simulink model "Lab8"  (R2015a)
settings: Solver=ode45  StartTime=0.0  StopTime=40  RelTol=1e-3
undefined symbols (not defined in the file or in its folder): currentCFG_Lab8_UB, fdesignblkfcn, gcbh, UB
libraries: dspstat3 x2, gtecHighspeedLib x1, gUSBamplib x1
settings Model: Creator=circuit  LastModifiedBy=circuit

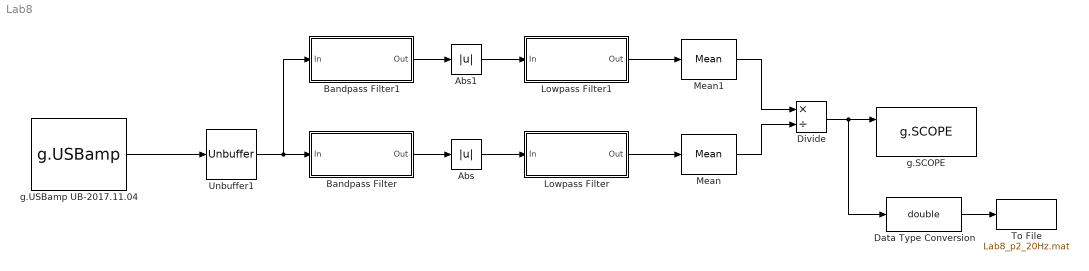
== system Lab8 ==
  Abs : Abs
  Abs1 : Abs
  Bandpass Filter : Subsystem  DialogController=fdesignblkfcn  InitFcn=fdesignblkfcn(gcbh, {'InitFcn'});  mask(Bandpass Filter){}
      mask help: Design a bandpass filter
      settings: CopyFcn=fdesignblkfcn(gcbh, {'CopyFcn'});
      mask Help: helpview(mapfilelocation('dsp'), 'dspbandpassfilter');
      mask Display: disp('Bandpass');
  Bandpass Filter1 : Subsystem  DialogController=fdesignblkfcn  InitFcn=fdesignblkfcn(gcbh, {'InitFcn'});  mask(Bandpass Filter){}
      mask help: Design a bandpass filter
      settings: CopyFcn=fdesignblkfcn(gcbh, {'CopyFcn'});
      mask Help: helpview(mapfilelocation('dsp'), 'dspbandpassfilter');
      mask Display: disp('Bandpass');
  Data Type Conversion : DataTypeConversion  OutDataTypeStr=double
  Divide : Product  Inputs=*/
  Lowpass Filter : Subsystem  DialogController=fdesignblkfcn  InitFcn=fdesignblkfcn(gcbh, {'InitFcn'});  mask(Lowpass Filter){}
      mask help: Design a lowpass filter
      settings: CopyFcn=fdesignblkfcn(gcbh, {'CopyFcn'});
      mask Help: helpview(mapfilelocation('dsp'), 'dsplowpassfilter');
      mask Display: disp('Lowpass')
  Lowpass Filter1 : Subsystem  DialogController=fdesignblkfcn  InitFcn=fdesignblkfcn(gcbh, {'InitFcn'});  mask(Lowpass Filter){}
      mask help: Design a lowpass filter
      settings: CopyFcn=fdesignblkfcn(gcbh, {'CopyFcn'});
      mask Help: helpview(mapfilelocation('dsp'), 'dsplowpassfilter');
      mask Display: disp('Lowpass')
  Mean : dspstat3/Mean  run=off  reset_popup=None  InputProcessing=Columns as channels (frame based)  directionMode=Each row  dimension=1  treatSBRowAsCol=off  roiEnable=off  roiType=Rectangles  roiPortion=Entire ROI  roiOutput=Individual statistics for each ROI  roiFlag=off  outputDataTypeStr=Inherit: Same as accumulator  outputLastDataTypeStr=Inherit: Same as accumulator  outputMin=[]  outputMax=[]  roundingMode=Floor  overflowMode=off
  Mean1 : dspstat3/Mean  run=off  reset_popup=None  InputProcessing=Columns as channels (frame based)  directionMode=Each row  dimension=1  treatSBRowAsCol=off  roiEnable=off  roiType=Rectangles  roiPortion=Entire ROI  roiOutput=Individual statistics for each ROI  roiFlag=off  outputDataTypeStr=Inherit: Same as accumulator  outputLastDataTypeStr=Inherit: Same as accumulator  outputMin=[]  outputMax=[]  roundingMode=Floor  overflowMode=off
  To File : ToFile  Filename=Lab8_p2_20Hz.mat
  Unbuffer1 : Unbuffer  SampleBasedProcessing=Same as frame based
  g.SCOPE : gtecHighspeedLib/g.SCOPE
  g.USBamp UB-2017.11.04 : gUSBamplib/g.USBamp  cfg=currentCFG_Lab8_UB-2017.11.04.cfg  snr=UB-2017.11.04
  wires:
  g.USBamp UB-2017.11.04/1 -> Unbuffer1/1
  Data Type Conversion/1 -> To File/1
  Bandpass Filter/1(Out) -> Abs/1
  Abs/1 -> Lowpass Filter/1(In)
  Lowpass Filter/1(Out) -> Mean/1
  Bandpass Filter1/1(Out) -> Abs1/1
  Abs1/1 -> Lowpass Filter1/1(In)
  Lowpass Filter1/1(Out) -> Mean1/1
  Unbuffer1/1 -> Bandpass Filter1/1(In), Bandpass Filter/1(In)
  Mean1/1 -> Divide/1
  Mean/1 -> Divide/2
  Divide/1 -> Data Type Conversion/1, g.SCOPE/1

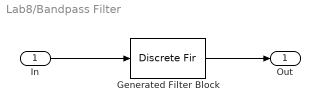
== system Lab8/Bandpass Filter ==
  In : Inport
  Generated Filter Block : DiscreteFir  Tag=BlockMethodSubSystem  Coefficients=[-9.707325903234668e-20 -1.4547940133680366e-05 -3.8949317559313134e-06 3.6026346384903206e-05 8.0448494737471273e-05 8.967465436443488e-05 3.7220119308981178e-05 -6.5501979123452491e-05 -0.00016597972781469807 -0.00019559147132576537 -0.00011199693878070027 6.5444622755014026e-05 0.00025203975411325575 0.00033537692656571258 0.00023929136553389044 -2.0493259905462968e-05 -0.00032560178590533242 -0.00050507650455621823 -0.0004277162252905762 -8.8528512668217872e-05 0.0003643080739927531 0.00068914948173672778 0.0006767539903635159 0.00027840235241952403 -0.00033958389430201825 -0.00085892159233023652 -0.00097081207789280141 -0.00055532890114523049 0.00022376136587924606 0.00097550797468224401 0.0012763435998424657 0.00090701727469001019 -1.3887637912025664e-18 -0.00099759244566786465 -0.0015439245373024095 -0.0012977059666992453 -0.00032731489556745731 0.00089308971486456654 0.0017161379540980648 0.0016685062324890048 0.00072466657028648004 -0.00065239693882807395 -0.001740671604790883 -0.0019445085536974286 -0.0011269354766907974 0.00030000334130668839 0.0015865019927581324 0.0020486066922622411 0.0014425109771110652 9.9042847240027109e-05 -0.0012597855387530821 -0.001920268606546659 -0.0015666716493755515 -0.00044075704605277499 0.00081544817158235193 0.0015359045645405192 0.0014020487983387941 0.0005935236471211751 -0.00036069024969694979 -0.00092644253770405118 -0.00088309532029252587 -0.00041873516814926295 4.776277178711424e-05 0.00018752915637505508 -6.5524449846833991e-19 -0.00020174488467054801 -5.5280066024992317e-05 0.00052141907608394336 0.0011832002845955873 0.0013357303032482299 0.00055968338192752905 -0.00099134229557729038 -0.0025212044943446008 -0.0029741453706790088 -0.0017007993626627198 0.0009904502538131809 0.003794183319845532 0.0050136260215938302 0.0035472478609025683 -0.00030087848750407051 -0.0047297848643821708 -0.0072531961505064354 -0.0060683103227048207 -0.0012403120709677583 0.0050386817714201193 0.0094078452364920653 0.0091185003577514967 0.0037027406841594478 -0.0044591076744620213 -0.0111389632161377 -0.0124394403636592 -0.0070342200886887255 0.0028035980128727342 0.012098431295184965 0.015680955581780381 0.011048464396676115 -1.5748967504052466e-17 -0.0119803203801235 -0.018439990783413261 -0.015432981404860749 -0.0038809415095607193 0.010572188456240368 0.02031262760549268 0.019777907844435092 0.008617426673178389 -0.0077973328141100204 -0.020951765911774806 -0.023622932270838583 -0.013850965299664677 0.0037402480337457382 0.020121480748256981 0.026516109949488494 0.019122696977364507 0.0013501128300229541 -0.017739032099786174 -0.028075943326947808 -0.023927330542281085 -0.0070812382767018274 0.013897069150475779 0.028047071501226335 0.027777174728241 0.012960135759938648 -0.0088615165124812691 -0.026340528101279799 -0.030266721377044666 -0.01845284220300266 0.0030444728151259146 0.023051734501646579 0.031127815551427521 0.023051734501646579 0.0030444728151259146 -0.01845284220300266 -0.030266721377044666 -0.026340528101279799 -0.0088615165124812691 0.012960135759938648 0.027777174728241 0.028047071501226335 0.013897069150475779 -0.0070812382767018274 -0.023927330542281085 -0.028075943326947808 -0.017739032099786174 0.0013501128300229541 0.019122696977364507 0.026516109949488494 0.020121480748256981 0.0037402480337457382 -0.013850965299664677 -0.023622932270838583 -0.020951765911774806 -0.0077973328141100204 0.008617426673178389 0.019777907844435092 0.02031262760549268 0.010572188456240368 -0.0038809415095607193 -0.015432981404860749 -0.018439990783413261 -0.0119803203801235 -1.5748967504052466e-17 0.011048464396676115 0.015680955581780381 0.012098431295184965 0.0028035980128727342 -0.0070342200886887255 -0.0124394403636592 -0.0111389632161377 -0.0044591076744620213 0.0037027406841594478 0.0091185003577514967 0.0094078452364920653 0.0050386817714201193 -0.0012403120709677583 -0.0060683103227048207 -0.0072531961505064354 -0.0047297848643821708 -0.00030087848750407051 0.0035472478609025683 ...(+1800 chars)]  InputProcessing=Columns as channels (frame based)
  Out : Outport
  wires:
  In/1 -> Generated Filter Block/1
  Generated Filter Block/1 -> Out/1

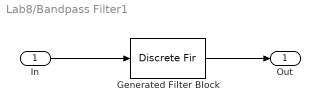
== system Lab8/Bandpass Filter1 ==
  In : Inport
  Generated Filter Block : DiscreteFir  Tag=BlockMethodSubSystem  Coefficients=[-1.5051096604374551e-18 -1.7315578160519554e-05 -2.2076592085780425e-05 -5.9277570357802236e-06 3.1389101425903213e-05 8.0816571350543964e-05 0.00012575429528274929 0.00014660285843847034 0.00012703399144143099 6.0301569398176467e-05 -4.6350086138402551e-05 -0.00017086650482735775 -0.0002800485001784454 -0.00033741029355496003 -0.00031362456545468598 -0.00019687808908326084 1.4905324401675337e-19 0.00023837594061658335 0.00046005735672647371 0.00060042917678830088 0.00060581554561807362 0.00045069373740795371 0.00014970350763937406 -0.00023988567888102094 -0.00062746234129258172 -0.00090922283468534656 -0.00099499177096056251 -0.00083498939690683494 -0.00043891889687715094 0.00011904202866567846 0.00071252172555333847 0.0011911226079923925 0.0014183952150465735 0.001310068670967178 0.00086189939415892843 0.0001583601107287249 -0.00064204422568400602 -0.0013428446473082586 -0.0017588812305126885 -0.0017662193847963654 -0.0013389945473798743 -0.00056213850641189137 0.00038505076969768689 0.0012716803113296596 0.0018740046664499222 0.0020347202706273528 0.0017064630006349019 0.00096686055046356085 4.7167813563242699e-19 -0.00095150144935152734 -0.0016511238977470455 -0.001931911061604685 -0.0017407731856561217 -0.0011507533051109246 -0.00033747433997506014 0.00047352502161691326 0.0010730699308501433 0.0013283913613479736 0.0012186513371829463 0.00083492833043168199 0.00034456292399080029 -6.8898475371502717e-05 -0.00027072084845249062 -0.00022320519157696217 1.0159490207952821e-17 0.0002401253570538214 0.00031332910165891191 8.5794034283249131e-05 -0.00046165678875068381 -0.0012037865562195325 -0.0018909823660554306 -0.0022187667634999313 -0.0019296252281738834 -0.00091693994760927281 0.00070387814007949164 0.0025859232729928535 0.0042158244117606637 0.005044023287598759 0.004649160935888701 0.0028905299566458318 -6.1862575527630841e-18 -0.0034232189366494221 -0.0065271566561753121 -0.0084122000165389298 -0.0083789297148803999 -0.0061525939479847936 -0.0020170867219165564 0.0031904703930140648 0.0082392663151604918 0.01179129713499929 0.012749265361490748 0.010576613566215332 0.0054993950464226771 -0.0014763813750679733 -0.0087539292168930267 -0.014509178704427236 -0.017146489245542868 -0.015732920258474781 -0.010294166910702493 -0.0018832992271464884 0.0076126571695153385 0.015896282806201065 0.020818547455569731 0.02093616646157033 0.015922753720059173 0.0067185799951697493 -0.004634701668396482 -0.015449054110653117 -0.023033061025488955 -0.025367579101915647 -0.021642936833123023 -0.012514545011860622 2.0009016392482179e-17 0.012970490553867205 0.023249465025490752 0.028246165819405887 0.02658633379172666 0.018488095480649051 0.0057513210558115466 -0.0086470152153513141 -0.021259496103246931 -0.029006649472020942 -0.029940091134921017 -0.023738604668124344 -0.011809359394900725 0.0030362214372321541 0.017256164848954109 0.027437156520506573 0.031127474356984049 0.027437156520506573 0.017256164848954109 0.0030362214372321541 -0.011809359394900725 -0.023738604668124344 -0.029940091134921017 -0.029006649472020942 -0.021259496103246931 -0.0086470152153513141 0.0057513210558115466 0.018488095480649051 0.02658633379172666 0.028246165819405887 0.023249465025490752 0.012970490553867205 2.0009016392482179e-17 -0.012514545011860622 -0.021642936833123023 -0.025367579101915647 -0.023033061025488955 -0.015449054110653117 -0.004634701668396482 0.0067185799951697493 0.015922753720059173 0.02093616646157033 0.020818547455569731 0.015896282806201065 0.0076126571695153385 -0.0018832992271464884 -0.010294166910702493 -0.015732920258474781 -0.017146489245542868 -0.014509178704427236 -0.0087539292168930267 -0.0014763813750679733 0.0054993950464226771 0.010576613566215332 0.012749265361490748 0.01179129713499929 0.0082392663151604918 0.0031904703930140648 -0.0020170867219165564 -0.0061525939479847936 -0.0083789297148803999 -0.0084122000165389298 -0.0065271566561753121 -0.0034232189366494221 -6.1862575527630841e-18 0.0028905299566458318 ...(+1821 chars)]  InputProcessing=Columns as channels (frame based)
  Out : Outport
  wires:
  In/1 -> Generated Filter Block/1
  Generated Filter Block/1 -> Out/1

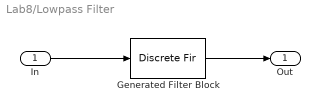
== system Lab8/Lowpass Filter ==
  In : Inport
  Generated Filter Block : DiscreteFir  Tag=BlockMethodSubSystem  Coefficients=[-2.426860513626208e-20 -2.4422383460267943e-06 -4.9085944088028271e-06 -7.4042474408730812e-06 -9.9344317405714216e-06 -1.2504424169548375e-05 -1.51195314397744e-05 -1.77850771864889e-05 -2.0506388843962146e-05 -2.3288784341308866e-05 -2.6137558635950667e-05 -2.9057970102656866e-05 -3.2055226796407254e-05 -3.5134472607611377e-05 -3.830077332848903e-05 -4.1559102649663359e-05 -4.4914328106241819e-05 -4.8371196992860719e-05 -5.1934322267348354e-05 -5.560816846281023e-05 -5.9397037628074024e-05 -6.3305055316532297e-05 -6.7336156643502349e-05 -7.1494072432276462e-05 -7.5782315469064961e-05 -8.0204166887039337e-05 -8.4762662699659782e-05 -8.9460580503426403e-05 -9.4300426370118291e-05 -9.9284421948490627e-05 -0.00010441449179526991 -0.00010969225095514504 -0.0001151189928092722 -0.00012069567721161313 -0.00012642291893220125 -0.00013230097642617873 -0.00013832974094717191 -0.00014450872602327449 -0.00015083705731357952 -0.00015731346286285592 -0.00016393626377159267 -0.00017070336529823404 -0.00017761224841001498 -0.00018465996179836111 -0.00019184311437435442 -0.00019915786825928065 -0.0002065999322847659 -0.00021416455601648351 -0.0002218465243148636 -0.00022964015244566994 -0.00023753928175272113 -0.0002455372759044314 -0.00025362701772521743 -0.00026180090662218306 -0.00027005085661683452 -0.00027836829499090782 -0.00028674416155469992 -0.00029516890854560014 -0.0003036325011637956 -0.00031212441875140448 -0.00032063365662054631 -0.00032914872853511318 -0.00033765766985023956 -0.0003461480413127076 -0.00035460693352473569 -0.00036302097207282683 -0.0003713763233225465 -0.00037965870087931542 -0.00038785337271449231 -0.00039594516895521796 -0.00040391849033568706 -0.00041175731730669585 -0.00041944521979951003 -0.00042696536763928139 -0.00043430054160243183 -0.00044143314511161562 -0.00044834521656106704 -0.00045501844226433243 -0.00046143417001559751 -0.00046757342325502406 -0.00047341691582772778 -0.00047894506732525159 -0.00048413801899762309 -0.00048897565022332625 -0.00049343759552376626 -0.00049750326210807889 -0.00050115184793340147 -0.00050436236026502057 -0.0005071136347201135 -0.000509384354778118 -0.00051115307174009941 -0.00051239822511884171 -0.00051309816344075011 -0.00051323116544004779 -0.00051277546162515329 -0.00051170925619655242 -0.00051001074929492968 -0.00050765815955778563 -0.00050462974696227126 -0.00050090383593146947 -0.00049645883868090833 -0.00049127327878163685 -0.00048532581491579564 -0.0004785952648002161 -0.00047106062925322698 -0.00046270111637951121 -0.00045349616584754225 -0.00044342547323385684 -0.00043246901440816156 -0.00042060706993304994 -0.00040782024945190589 -0.00039408951603841152 -0.0003793962104809249 -0.0003637220754749031 -0.00034704927969645121 -0.00032936044173003916 -0.00031063865382340803 -0.00029086750544269583 -0.00027003110660086117 -0.00024811411093255233 -0.00022510173848867165 -0.00020097979822402402 -0.00017573471015159937 -0.00014935352713722983 -0.00012182395630859965 -9.313438005282834e-05 -6.327387657713907e-05 -3.2232240007442718e-05 1.6381308466976901e-19 3.3431559158283158e-05 6.8070379984983952e-05 0.00010392361379633834 0.00014099760328361595 0.00017929786569438082 0.00021882907664078262 0.00025959505455650563 0.00030159874582342053 0.00034484221058839209 0.00038932660929008958 0.00043505218991497709 0.00048201827600102311 0.00053022325540695602 0.00057966456986419199 0.00063033870532781323 0.00068224118314224138 0.00073536655203644042 0.00078970838096272086 0.0008452592527923797 0.00090201075888058236 0.00095995349451206155 0.0010190770552383048 0.0010793700341160566 0.0011408200198560513 0.0012034135958899795 0.0012671363403627784 0.0013319728270564076 0.0013979066272503081 0.0014649203125228203 0.0015329954584968515 0.0016021126495321275 0.0016722514843653983 0.0017433905826989581 0.001815507592736898 0.001888579199667487 0.0019625811350891158 0.0020374881873762378 0.0021132742129807507 0.0021899121486632744 0.0022673740246478228 0.0023456309786923325 ...(+7779 chars)]  InputProcessing=Columns as channels (frame based)
  Out : Outport
  wires:
  In/1 -> Generated Filter Block/1
  Generated Filter Block/1 -> Out/1

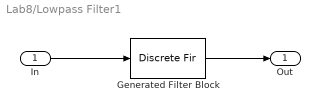
== system Lab8/Lowpass Filter1 ==
  In : Inport
  Generated Filter Block : DiscreteFir  Tag=BlockMethodSubSystem  Coefficients=[-2.426860513626208e-20 -2.4422383460267943e-06 -4.9085944088028271e-06 -7.4042474408730812e-06 -9.9344317405714216e-06 -1.2504424169548375e-05 -1.51195314397744e-05 -1.77850771864889e-05 -2.0506388843962146e-05 -2.3288784341308866e-05 -2.6137558635950667e-05 -2.9057970102656866e-05 -3.2055226796407254e-05 -3.5134472607611377e-05 -3.830077332848903e-05 -4.1559102649663359e-05 -4.4914328106241819e-05 -4.8371196992860719e-05 -5.1934322267348354e-05 -5.560816846281023e-05 -5.9397037628074024e-05 -6.3305055316532297e-05 -6.7336156643502349e-05 -7.1494072432276462e-05 -7.5782315469064961e-05 -8.0204166887039337e-05 -8.4762662699659782e-05 -8.9460580503426403e-05 -9.4300426370118291e-05 -9.9284421948490627e-05 -0.00010441449179526991 -0.00010969225095514504 -0.0001151189928092722 -0.00012069567721161313 -0.00012642291893220125 -0.00013230097642617873 -0.00013832974094717191 -0.00014450872602327449 -0.00015083705731357952 -0.00015731346286285592 -0.00016393626377159267 -0.00017070336529823404 -0.00017761224841001498 -0.00018465996179836111 -0.00019184311437435442 -0.00019915786825928065 -0.0002065999322847659 -0.00021416455601648351 -0.0002218465243148636 -0.00022964015244566994 -0.00023753928175272113 -0.0002455372759044314 -0.00025362701772521743 -0.00026180090662218306 -0.00027005085661683452 -0.00027836829499090782 -0.00028674416155469992 -0.00029516890854560014 -0.0003036325011637956 -0.00031212441875140448 -0.00032063365662054631 -0.00032914872853511318 -0.00033765766985023956 -0.0003461480413127076 -0.00035460693352473569 -0.00036302097207282683 -0.0003713763233225465 -0.00037965870087931542 -0.00038785337271449231 -0.00039594516895521796 -0.00040391849033568706 -0.00041175731730669585 -0.00041944521979951003 -0.00042696536763928139 -0.00043430054160243183 -0.00044143314511161562 -0.00044834521656106704 -0.00045501844226433243 -0.00046143417001559751 -0.00046757342325502406 -0.00047341691582772778 -0.00047894506732525159 -0.00048413801899762309 -0.00048897565022332625 -0.00049343759552376626 -0.00049750326210807889 -0.00050115184793340147 -0.00050436236026502057 -0.0005071136347201135 -0.000509384354778118 -0.00051115307174009941 -0.00051239822511884171 -0.00051309816344075011 -0.00051323116544004779 -0.00051277546162515329 -0.00051170925619655242 -0.00051001074929492968 -0.00050765815955778563 -0.00050462974696227126 -0.00050090383593146947 -0.00049645883868090833 -0.00049127327878163685 -0.00048532581491579564 -0.0004785952648002161 -0.00047106062925322698 -0.00046270111637951121 -0.00045349616584754225 -0.00044342547323385684 -0.00043246901440816156 -0.00042060706993304994 -0.00040782024945190589 -0.00039408951603841152 -0.0003793962104809249 -0.0003637220754749031 -0.00034704927969645121 -0.00032936044173003916 -0.00031063865382340803 -0.00029086750544269583 -0.00027003110660086117 -0.00024811411093255233 -0.00022510173848867165 -0.00020097979822402402 -0.00017573471015159937 -0.00014935352713722983 -0.00012182395630859965 -9.313438005282834e-05 -6.327387657713907e-05 -3.2232240007442718e-05 1.6381308466976901e-19 3.3431559158283158e-05 6.8070379984983952e-05 0.00010392361379633834 0.00014099760328361595 0.00017929786569438082 0.00021882907664078262 0.00025959505455650563 0.00030159874582342053 0.00034484221058839209 0.00038932660929008958 0.00043505218991497709 0.00048201827600102311 0.00053022325540695602 0.00057966456986419199 0.00063033870532781323 0.00068224118314224138 0.00073536655203644042 0.00078970838096272086 0.0008452592527923797 0.00090201075888058236 0.00095995349451206155 0.0010190770552383048 0.0010793700341160566 0.0011408200198560513 0.0012034135958899795 0.0012671363403627784 0.0013319728270564076 0.0013979066272503081 0.0014649203125228203 0.0015329954584968515 0.0016021126495321275 0.0016722514843653983 0.0017433905826989581 0.001815507592736898 0.001888579199667487 0.0019625811350891158 0.0020374881873762378 0.0021132742129807507 0.0021899121486632744 0.0022673740246478228 0.0023456309786923325 ...(+7779 chars)]  InputProcessing=Columns as channels (frame based)
  Out : Outport
  wires:
  In/1 -> Generated Filter Block/1
  Generated Filter Block/1 -> Out/1
